simulink model "Load_torque_1st_order_estimator"  (R2021a)
settings: Solver=FixedStepDiscrete  StartTime=0.0  StopTime=10.0  FixedStep=1e-5  RelTol=1e-3
undefined symbols (not defined in the file): DiscIntNeverNeededParam
settings Model: Creator=Mehra  LastModifiedBy=Mehra

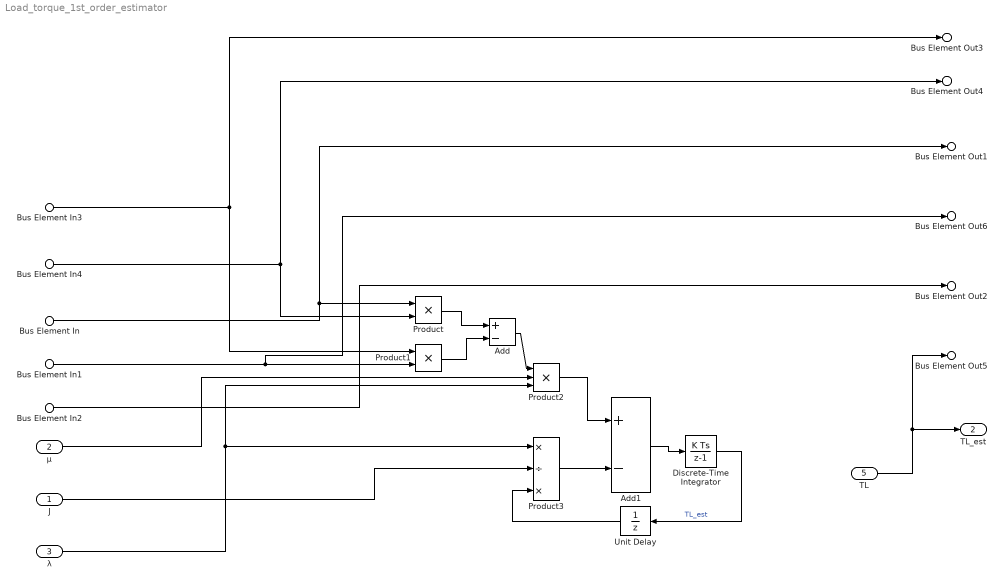
== system Load_torque_1st_order_estimator ==
  J : Inport
  µ : Inport  Port=2
  λ : Inport  Port=3
  Bus Element In4 : Inport  Port=4  PortName=mesin  Element=Isb
  Bus Element In3 : Inport  Port=4  PortName=mesin  Element=Isa
  Bus Element In : Inport  Port=4  PortName=mesin  Element=Ψra
  Bus Element In1 : Inport  Port=4  PortName=mesin  Element=Ψrb
  Bus Element In2 : Inport  Port=4  PortName=mesin  Element=ω
  TL : Inport  Port=5
  Add : Sum  Inputs=+-
  Add1 : Sum  Inputs=+-
  Discrete-Time Integrator : DiscreteIntegrator  SampleTime=-1  ICPrevOutput=DiscIntNeverNeededParam  ICPrevScaledInput=DiscIntNeverNeededParam
  Product : Product
  Product1 : Product
  Product2 : Product  Inputs=3
  Product3 : Product  Inputs=*/*
  Unit Delay : UnitDelay  SampleTime=-1  HasFrameUpgradeWarning=on
  Bus Element Out2 : Outport  PortName=mes  Element=ω
  Bus Element Out3 : Outport  PortName=mes  Element=Isa
  Bus Element Out4 : Outport  PortName=mes  Element=Isb
  Bus Element Out5 : Outport  PortName=mes  Element=TL
  Bus Element Out1 : Outport  PortName=mes  Element=Ψra
  Bus Element Out6 : Outport  PortName=mes  Element=Ψrb
  TL_est : Outport  Port=2
  wires:
  Product/1 -> Add/1
  Bus Element In1/1 -> Bus Element Out6/1, Product1/2
  Product1/1 -> Add/2
  Product3/1 -> Add1/2
  Bus Element In3/1 -> Bus Element Out3/1, Product1/1
  Add/1 -> Product2/1
  J/1 -> Product3/2
  Bus Element In4/1 -> Product/2, Bus Element Out4/1
  Bus Element In/1 -> Bus Element Out1/1, Product/1
  µ/1 -> Product2/2
  Add1/1 -> Discrete-Time Integrator/1
  Product2/1 -> Add1/1
  Discrete-Time Integrator/1 -> Unit Delay/1  "TL_est"
  λ/1 -> Product3/1, Product2/3
  Unit Delay/1 -> Product3/3
  Bus Element In2/1 -> Bus Element Out2/1
  TL/1 -> TL_est/1, Bus Element Out5/1
